simulink model "be2"  (R2013a)
settings: Solver=ode45  StartTime=0.0  StopTime=10.0  RelTol=1e-3
values from neighbouring files (symbols this model uses):
  A = -f0/J    (= -4.5652173913)    [variablesCC.m]
  B = Km/J    (= 652.173913043)    [variablesCC.m]
  C = 1    [variablesCC.m]
  f1 = 1.5 * 10^(-4)    (= 0.00015)    [variablesCC.m]
  g2 = 1/(-C*(A-B*Kt)^(-1)*B)    [variablesCC.m]
  J = 9.2 * 10^(-5)    (= 9.2e-05)    [variablesCC.m]
  Kr = Kinterm(2)    [variablesCC.m]
  Kt = Kinterm(1)    [variablesCC.m]
settings Model: Creator=tfumey  LastModifiedBy=tfumey

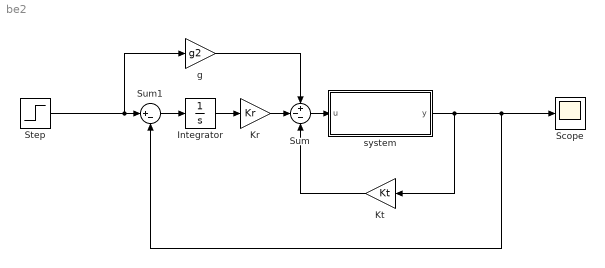
== system be2 ==
  Integrator : Integrator
  Kr : Gain  Gain=Kr
  "Kt " : Gain  Gain=Kt
  Scope : Scope
  Step : Step  SampleTime=0
  Sum : Sum  Inputs=+--
  Sum1 : Sum  Inputs=|+-
  g : Gain  Gain=g2
  system : Subsystem
  wires:
  Kr/1 -> Sum/2
  Sum/1 -> system/1(u)
  Step/1 -> g/1, Sum1/1
  system/1(y) -> "Kt "/1, Sum1/2, Scope/1
  "Kt "/1 -> Sum/3
  Integrator/1 -> Kr/1
  Sum1/1 -> Integrator/1
  g/1 -> Sum/1

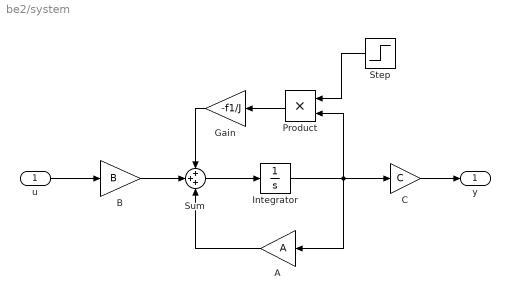
== system be2/system ==
  u : Inport
  A : Gain  Gain=A
  B : Gain  Gain=B
  C : Gain  Gain=C
  Gain : Gain  Gain=-f1/J
  Integrator : Integrator
  Product : Product
  Step : Step  Time=1.1  SampleTime=0
  Sum : Sum  Inputs=+++
  y : Outport
  wires:
  u/1 -> B/1
  Sum/1 -> Integrator/1
  Integrator/1 -> Product/2, C/1, A/1
  C/1 -> y/1
  A/1 -> Sum/3
  B/1 -> Sum/2
  Gain/1 -> Sum/1
  Product/1 -> Gain/1
  Step/1 -> Product/1
